simulink model "svpwm_speed"  (R2024b)
settings: Solver=VariableStepAuto  StartTime=0.0  StopTime=inf  RelTol=1e-3
libraries: simulink x2, spsDCVoltageSourceLib x1, spsPermanentMagnetSynchronousMachineLib x1, sldrtlib x1, spsTwoLevelConverterLib x1, spspowerguiLib x1
settings Model: Creator=alienware  LastModifiedBy=20844

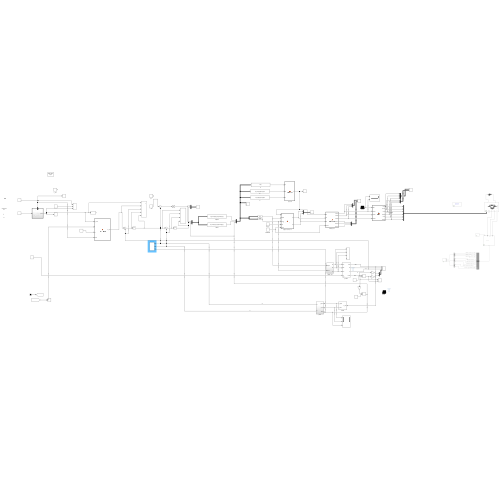
[thumbnail: Simulink's stored preview of the top-level diagram]
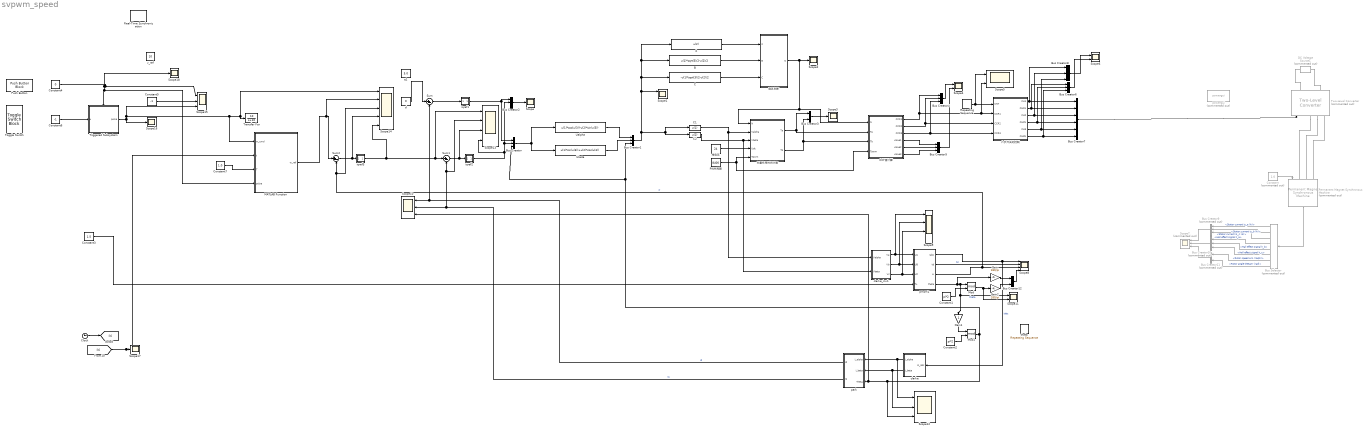
== system svpwm_speed ==
  A : Fcn  Expr=u(2)
  B : Fcn  Expr=u(1)*sqrt(3)/2-u(2)/2
  Bus Creator{,1..2,4..6,8} (7 alike) : BusCreator  Inputs=3
  Bus Creator10 : BusCreator  Commented=on  Inputs=3
  Bus Creator11 : BusCreator  Commented=on  Inputs=2
  Bus Creator12 : BusCreator  Inputs=2
  Bus Creator3 : BusCreator  Inputs=2
  Bus Creator7 : BusCreator  Inputs=6
  Bus Creator9 : BusCreator  Commented=on  Inputs=3
  Bus Selector : BusSelector  Commented=on  OutputSignals=Stator current is_a (A),Stator current is_b (A),Stator current is_c (A),Hall effect signal h_a,Hall effect signal h_b,Hall effect signal h_c,Rotor speed wm (rad/s),Rotor angle thetam (rad)
  C : Fcn  Expr=-u(1)*sqrt(3)/2-u(2)/2
  C1 : Fcn  Expr=u(1)
  C2 : Fcn  Expr=u(2)
  CCR值计算 : MATLAB Function  TreatAsAtomicUnit=on
  Clock : Clock
  Constant : Constant  Commented=on  Value=1.0
  Constant1 : Constant  Value=pi*2
  Constant2 : Constant  Value=pi*2
  Constant3 : Constant  Value=1.5
  Constant4 : Constant  Value=0
  Constant5 : Constant  Value=-1
  Constant6 : Constant  Value=-1
  Constant7 : Constant  Value=1.0
  DC Voltage Source1 : spsDCVoltageSourceLib/DC Voltage Source  Commented=on  Amplitude=24  Measurements=None
  Gain : Gain  Gain=180/pi
  Gain1 : Gain
  Gain2 : Gain  Gain=180/pi
  MATLAB Function : MATLAB Function  TreatAsAtomicUnit=on
  Mod : Math  Operator=mod
  Mod1 : Math  Operator=mod
  PWM周期 : Constant  Value=8400
  Permanent Magnet Synchronous Machine : spsPermanentMagnetSynchronousMachineLib/Permanent Magnet Synchronous Machine  Commented=on  NbPhases=3  FluxDistribution=Sinusoidal  RotorType=Round  MechanicalLoad=Torque Tm  PresetModel=No  ShowDetailedParameters=on  MeasurementBus=off  Resistance=0.0485  Inductance=8.5e-3  dqInductances=[8.5e-3,8.5e-3]  La=0.000395  MachineConstant=Flux linkage established by magnets (V.s)  Flux=0.1194  VoltageCst=86.6271  TorqueCst=0.7164  Flat=120  Mechanical=[0.0027 0.0004924 4 0]  PolePairs=4  InitialConditions=[0,0, 0,0]  InitialConditions5ph=[0 0 0 0 0 0]  RefAngle=Aligned with phase A axis (original Park)  IterativeDiscreteModel=Trapezoidal non iterative  TsBlock=-1  TsPowergui=0
  Push Button : PushButtonBlock  OnValue=2  OffValue=0.000000
  Real-Time Synchronization : sldrtlib/Real-Time Synchronization  SampleTime=0.001  MaxMissedTicks=inf  ShowMissedTicks=off  YieldWhenWaiting=off
  Repeating Sequence : simulink/Sources/Repeating Sequence  rep_seq_t=[0 0.00005 0.0001]  rep_seq_y=[0 4200 0]
  Scope{,2..3,16..18} (6 alike) : Scope
  Scope{1,10,12,15} (4 alike) : Scope  NumInputPorts=3
  Scope{4..6,11} (4 alike) : Scope  NumInputPorts=2
  Scope13 : Scope  NumInputPorts=4
  Scope14 : Scope  NumInputPorts=5
  Scope7 : Scope  Commented=on  NumInputPorts=3
  Scope8 : Scope  NumInputPorts=4
  Scope9 : Scope  NumInputPorts=4
  Sum : Sum  Inputs=|+-
  Sum1 : Sum  Inputs=|+-
  Sum2 : Sum  Inputs=|+-
  Toggle Switch : ToggleSwitchBlock
      settings: Values={{'Off', 'On'}, [-1 1]}
  Transfer Fcn : TransferFcn  Numerator=[10]  Denominator=[1 10]
  Triggered Subsystem : Subsystem  TreatAsAtomicUnit=on
  Two-Level Converter : spsTwoLevelConverterLib/Two-Level Converter  Commented=on  ModelType=Switching devices  Ron=1e-3  Rs=1e6  Cs=inf  Vforward=[0,0]  Ron_Diode=1e-3  Rs_Diode=1e6  Cs_Diode=inf  Vf_Diode=1e-3  Rs_CurrentSource=inf  Ron_ACsource=1e-3
      settings: LibrarySourceBlock=sps_lib/Power Electronics/Two-Level Converter
  Ualpha : Fcn  Expr=u(1)*cos(u(3))-u(2)*sin(u(3))
  Ubeta : Fcn  Expr=u(1)*sin(u(3))+u(2)*cos(u(3))
  clarke : Subsystem
  clarke_inv1 : Subsystem
  d : Constant  Value=0
  iqref1 : Subsystem  mask(PI Controller){I=0, P=0, sat=[-500, 500]}
      mask prompts: I "Integral"; P "Proportional:"; sat "Minimum and maximum outputs:"
      mask init:
      | min=sat(1);max=sat(2);
      mask Display: disp('PI')
  iqref2 : Subsystem  mask(PI Controller){I=0, P=1, sat=[-500, 500]}
      mask prompts: I "Integral"; P "Proportional:"; sat "Minimum and maximum outputs:"
      mask init:
      | min=sat(1);max=sat(2);
      mask Display: disp('PI')
  iqref3 : Subsystem  mask(PI Controller){I=10, P=10, sat=[-100, 100]}
      mask prompts: I "Integral"; P "Proportional:"; sat "Minimum and maximum outputs:"
      mask init:
      | min=sat(1);max=sat(2);
      mask Display: disp('PI')
  park : Subsystem
  pmsm1 : Subsystem  mask(hao){CL=0.175, Pm=4, Ld=0.0085, Lq=0.0085, rs=2.875, J=0.0008}
      mask help: pmsm
      mask Help: no
  powergui : spspowerguiLib/powergui  Priority=1  Commented=on  SimulationMode=Discrete  SampleTime=0.000001  frequency=60  Iterations=50  frequencyindice=0  Pbase=100e6  ErrMax=1e-4  UnitsV=kV  UnitsW=MW  buscounter=0  FunctionMessages=off  echomessages=off  EnableUseOfTLC=off  CurrentSourceSwitches=off  DisableSnubberDevices=off  DisableRonSwitches=off  DisableVfSwitches=off  DisplayEquations=off  AutomaticDiscreteSolvers=off  SolverType=Tustin/Backward Euler (TBE)  Interpol=off  ExternalGateDelay=off  methode=off  Ts=100  x0status=blocks  SPID=on  SwTol=0  HookPort=off  NonlinearTolerance=1e-4  nMaxIteration=100  ContinueOnMaxIteration=off  RestoreLinks=warning  ResistiveCurrentMeasurement=off  Frange=[0:2:500]  Ylog=off  Xlog=on  ShowGrid=off  save=off  variable=ZData  structure=0  ZoomFFT=off  StartTime=0.0  cycles=1  DisplayStyle=1  fundamental=60  FreqAxis=off  MaxFrequency=1000  frequencyindicesteady=1  RmsSteady=1  display=off
  q1 : Constant  Value=5.0
  "theta " : simulink/Sources/Repeating Sequence  rep_seq_t=[0 1]  rep_seq_y=[0 2*pi]
  v_ref : Constant  Value=10
  六步开关的控制 : MATLAB Function  TreatAsAtomicUnit=on
  扇区判断 : MATLAB Function  TreatAsAtomicUnit=on
  矢量作用时间计算 : MATLAB Function  TreatAsAtomicUnit=on
  线电压 : Constant  Value=24
  wires:
  Sum/1 -> iqref1/1(In_1)
  Sum1/1 -> Scope13/3, iqref2/1(In_1)
  Bus Creator/1 -> Ubeta/1, Ualpha/1
  Ualpha/1 -> Bus Creator1/1
  Ubeta/1 -> Bus Creator1/2
  Bus Creator2/1 -> Scope/1
  Bus Creator1/1 -> A/1, B/1, C/1, Scope1/1, C1/1, C2/1
  A/1 -> 扇区判断/1(A)
  B/1 -> 扇区判断/2(B)
  C/1 -> 扇区判断/3(C)
  扇区判断/1(N) -> Scope2/1, CCR值计算/1(N), 矢量作用时间计算/1(N)
  C1/1 -> clarke_inv1/1(Valpha), 矢量作用时间计算/2(Valpha)
  C2/1 -> clarke_inv1/2(Vbeta), 矢量作用时间计算/3(Vbeta)
  线电压/1 -> 矢量作用时间计算/4(Udc)
  PWM周期/1 -> CCR值计算/4(Tpwm), 矢量作用时间计算/5(Tpwm)
  矢量作用时间计算/1(Ta) -> Bus Creator3/1, CCR值计算/2(Ta)
  矢量作用时间计算/2(Tb) -> Bus Creator3/2, CCR值计算/3(Tb)
  Bus Creator3/1 -> Scope3/1
  CCR值计算/3(CCR3) -> 六步开关的控制/4(CCR3), Bus Creator4/3
  CCR值计算/2(CCR2) -> Bus Creator4/2, 六步开关的控制/3(CCR2)
  CCR值计算/1(CCR1) -> Scope5/2, 六步开关的控制/2(CCR1), Bus Creator4/1
  Bus Creator4/1 -> Scope4/1
  CCR值计算/4(value1) -> Bus Creator5/1
  CCR值计算/5(value2) -> Bus Creator5/2
  CCR值计算/6(value3) -> Bus Creator5/3
  Bus Creator5/1 -> Scope4/2
  Repeating Sequence/1 -> 六步开关的控制/1(CNT), Scope5/1
  六步开关的控制/1(CH1) -> Bus Creator7/1, Bus Creator8/1
  六步开关的控制/2(CH1N) -> Bus Creator7/2, Bus Creator6/1
  六步开关的控制/3(CH2) -> Bus Creator7/3, Bus Creator8/2
  六步开关的控制/5(CH3) -> Bus Creator7/5, Bus Creator8/3
  六步开关的控制/4(CH2N) -> Bus Creator7/4, Bus Creator6/2
  六步开关的控制/6(CH3N) -> Bus Creator7/6, Bus Creator6/3
  Bus Creator8/1 -> Scope6/1
  Bus Creator7/1 -> Two-Level Converter/1
  Constant/1 -> Permanent Magnet Synchronous Machine/1
  Permanent Magnet Synchronous Machine/1 -> Bus Selector/1
  Bus Creator9/1 -> Scope7/1
  Bus Creator10/1 -> Scope7/2
  Bus Creator11/1 -> Scope7/3
  Bus Selector/1 -> Bus Creator9/1  "<Stator current is_a (A)>"
  Bus Selector/2 -> Bus Creator9/2  "<Stator current is_b (A)>"
  Bus Selector/3 -> Bus Creator9/3  "<Stator current is_c (A)>"
  Bus Selector/4 -> Bus Creator10/1  "<Hall effect signal h_a>"
  Bus Selector/5 -> Bus Creator10/2  "<Hall effect signal h_b>"
  Bus Selector/6 -> Bus Creator10/3  "<Hall effect signal h_c>"
  Bus Selector/7 -> Bus Creator11/1  "<Rotor speed wm (rad/s)>"
  Bus Selector/8 -> Bus Creator11/2  "<Rotor angle thetam (rad)>"
  Bus Creator6/1 -> Scope6/2
  clarke_inv1/1(Va) -> Scope9/1, pmsm1/1(UA)
  clarke_inv1/2(Vb) -> Scope9/2, pmsm1/2(UB)
  clarke_inv1/3(Vc) -> Scope9/3, pmsm1/3(UC)
  Constant3/1 -> pmsm1/4(TL)
  pmsm1/1(iabc) -> Scope8/1, clarke/1(is_abc)  "iabc"
  pmsm1/2(td) -> Scope8/2  "td"
  pmsm1/3(w) -> Scope8/3, Scope14/3, Sum2/2  "w"
  pmsm1/4(theta) -> Gain/1, Scope11/1, Gain1/1, Mod/1  "theta"
  Constant1/1 -> Mod/2
  Mod/1 -> Gain2/1, Scope11/2
  Gain/1 -> Bus Creator12/1
  clarke/1(I_alpha) -> park/1(I_alpha), Scope12/1
  clarke/2(I_beta) -> park/2(I_beta), Scope12/2
  park/1(Id) -> Sum/2, Scope10/1  "id"
  park/2(Iq) -> Scope13/2, Sum1/2, Scope10/2  "iq"
  Gain1/1 -> Mod1/1
  Constant2/1 -> Mod1/2
  Gain2/1 -> Bus Creator12/2
  Bus Creator12/1 -> Scope8/4
  d/1 -> Sum/1
  iqref3/1(Out_1) -> Scope14/5, Scope13/1, Sum1/1
  iqref1/1(Out_1) -> Bus Creator/1, Bus Creator2/1
  iqref2/1(Out_1) -> Scope13/4, Bus Creator2/2, Bus Creator/2
  Mod1/1 -> Bus Creator/3, Bus Creator1/3, Scope12/3, Scope10/3, park/3(Theta)
  Triggered Subsystem/1(pulse) -> Scope15/3, MATLAB Function/1(w_cmd), Transfer Fcn/1, Scope14/1, Scope16/1
  Sum2/1 -> Scope14/4, iqref3/1(In_1)
  Constant5/1 -> Scope15/2
  Constant6/1 -> Triggered Subsystem/1(u)
  MATLAB Function/1(w_ref) -> Scope14/2, Sum2/1
  Clock/1 -> [t]
  [t] -> MATLAB Function/2(t), Scope17/1
  Constant7/1 -> MATLAB Function/3(T)
  Constant4/1 -> MATLAB Function/4(pulse), Triggered Subsystem/Trigger, Scope18/1, Scope15/1
  connections:
  DC Voltage Source1/RConn1 -- Two-Level Converter/RConn1
  DC Voltage Source1/LConn1 -- Two-Level Converter/RConn2
  Permanent Magnet Synchronous Machine/LConn3 -- Two-Level Converter/LConn3
  Two-Level Converter/LConn2 -- Permanent Magnet Synchronous Machine/LConn2
  Two-Level Converter/LConn1 -- Permanent Magnet Synchronous Machine/LConn1

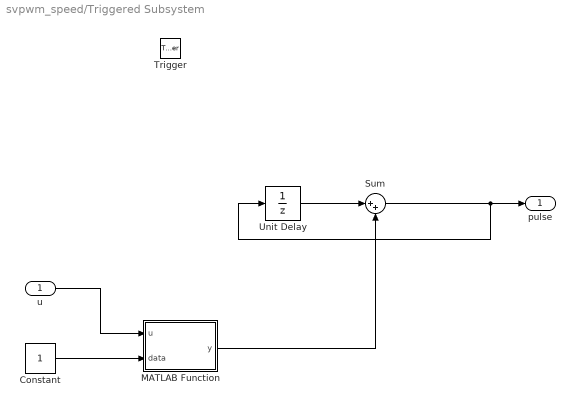
== system svpwm_speed/Triggered Subsystem ==
  u : Inport
  Trigger : TriggerPort  VariantControl=(inherit)
  Constant : Constant
  MATLAB Function : MATLAB Function  TreatAsAtomicUnit=on
  Sum : Sum  Inputs=|++
  Unit Delay : UnitDelay  InitialCondition=10  InputProcessing=Columns as channels (frame based)  SampleTime=-1  HasFrameUpgradeWarning=on
  pulse : Outport
  wires:
  Unit Delay/1 -> Sum/1
  MATLAB Function/1(y) -> Sum/2
  Sum/1 -> Unit Delay/1, pulse/1
  u/1 -> MATLAB Function/1(u)
  Constant/1 -> MATLAB Function/2(data)

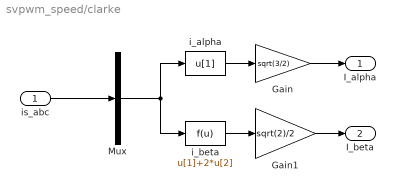
== system svpwm_speed/clarke ==
  is_abc : Inport
  Gain : Gain  Gain=sqrt(3/2)  SaturateOnIntegerOverflow=on  OutDataTypeStr=Inherit: Same as input  ParamDataTypeStr=Inherit: Same as input
  Gain1 : Gain  Gain=sqrt(2)/2  SaturateOnIntegerOverflow=on  OutDataTypeStr=Inherit: Same as input  ParamDataTypeStr=Inherit: Same as input
  Mux : Mux  Inputs=[3]
  i_alpha : Fcn  Expr=u[1]
  i_beta : Fcn  Expr=u[1]+2*u[2]
  I_alpha : Outport  InitialOutput=0
  I_beta : Outport  Port=2  InitialOutput=0
  wires:
  Mux/1 -> i_beta/1, i_alpha/1
  is_abc/1 -> Mux/1
  i_beta/1 -> Gain1/1
  i_alpha/1 -> Gain/1
  Gain/1 -> I_alpha/1
  Gain1/1 -> I_beta/1

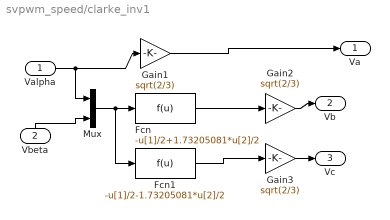
== system svpwm_speed/clarke_inv1 ==
  Valpha : Inport
  Vbeta : Inport  Port=2
  Fcn : Fcn  Expr=-u[1]/2+1.73205081*u[2]/2
  Fcn1 : Fcn  Expr=-u[1]/2-1.73205081*u[2]/2
  Gain1 : Gain  Gain=sqrt(2/3)  SaturateOnIntegerOverflow=on  OutDataTypeStr=Inherit: Same as input  ParamDataTypeStr=Inherit: Same as input
  Gain2 : Gain  Gain=sqrt(2/3)  SaturateOnIntegerOverflow=on  OutDataTypeStr=Inherit: Same as input  ParamDataTypeStr=Inherit: Same as input
  Gain3 : Gain  Gain=sqrt(2/3)  SaturateOnIntegerOverflow=on  OutDataTypeStr=Inherit: Same as input  ParamDataTypeStr=Inherit: Same as input
  Mux : Mux  Inputs=2
  Va : Outport
  Vb : Outport  Port=2
  Vc : Outport  Port=3
  wires:
  Gain3/1 -> Vc/1
  Gain2/1 -> Vb/1
  Gain1/1 -> Va/1
  Vbeta/1 -> Mux/2
  Valpha/1 -> Mux/1, Gain1/1
  Fcn1/1 -> Gain3/1
  Fcn/1 -> Gain2/1
  Mux/1 -> Fcn1/1, Fcn/1

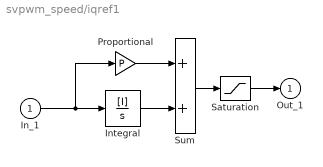
== system svpwm_speed/iqref1 ==
  In_1 : Inport
  Integral : TransferFcn  Numerator=[I]  Denominator=[1 0]
  Proportional : Gain  Gain=P  SaturateOnIntegerOverflow=on  OutDataTypeStr=Inherit: Same as input  ParamDataTypeStr=Inherit: Same as input
  Saturation : Saturate  UpperLimit=max  LowerLimit=min
  Sum : Sum  InputSameDT=on  SaturateOnIntegerOverflow=on  OutDataTypeStr=Inherit: Same as first input
  Out_1 : Outport  InitialOutput=0
  wires:
  Saturation/1 -> Out_1/1
  Sum/1 -> Saturation/1
  Proportional/1 -> Sum/1
  In_1/1 -> Proportional/1, Integral/1
  Integral/1 -> Sum/2

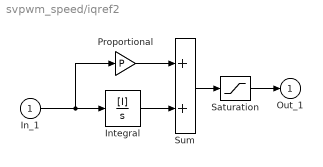
== system svpwm_speed/iqref2 ==
  In_1 : Inport
  Integral : TransferFcn  Numerator=[I]  Denominator=[1 0]
  Proportional : Gain  Gain=P  SaturateOnIntegerOverflow=on  OutDataTypeStr=Inherit: Same as input  ParamDataTypeStr=Inherit: Same as input
  Saturation : Saturate  UpperLimit=max  LowerLimit=min
  Sum : Sum  InputSameDT=on  SaturateOnIntegerOverflow=on  OutDataTypeStr=Inherit: Same as first input
  Out_1 : Outport  InitialOutput=0
  wires:
  Integral/1 -> Sum/2
  In_1/1 -> Integral/1, Proportional/1
  Proportional/1 -> Sum/1
  Sum/1 -> Saturation/1
  Saturation/1 -> Out_1/1

== system svpwm_speed/iqref3 ==
  In_1 : Inport
  Integral : TransferFcn  Numerator=[I]  Denominator=[1 0]
  Proportional : Gain  Gain=P  SaturateOnIntegerOverflow=on  OutDataTypeStr=Inherit: Same as input  ParamDataTypeStr=Inherit: Same as input
  Saturation : Saturate  UpperLimit=max  LowerLimit=min
  Sum : Sum  InputSameDT=on  SaturateOnIntegerOverflow=on  OutDataTypeStr=Inherit: Same as first input
  Out_1 : Outport  InitialOutput=0
  wires:
  Integral/1 -> Sum/2
  In_1/1 -> Integral/1, Proportional/1
  Proportional/1 -> Sum/1
  Sum/1 -> Saturation/1
  Saturation/1 -> Out_1/1

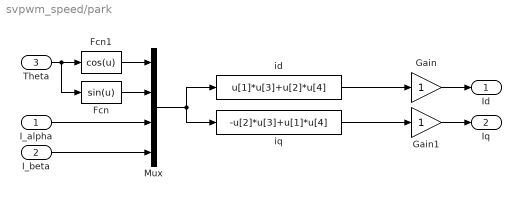
== system svpwm_speed/park ==
  I_alpha : Inport
  I_beta : Inport  Port=2
  Theta : Inport  Port=3
  Fcn : Fcn  Expr=sin(u)
  Fcn1 : Fcn  Expr=cos(u)
  Gain : Gain  SaturateOnIntegerOverflow=on  OutDataTypeStr=Inherit: Same as input  ParamDataTypeStr=Inherit: Same as input
  Gain1 : Gain  SaturateOnIntegerOverflow=on  OutDataTypeStr=Inherit: Same as input  ParamDataTypeStr=Inherit: Same as input
  Mux : Mux  Inputs=[1 1 1 1]
  id : Fcn  Expr=u[1]*u[3]+u[2]*u[4]
  iq : Fcn  Expr=-u[2]*u[3]+u[1]*u[4]
  Id : Outport  InitialOutput=0
  Iq : Outport  Port=2  InitialOutput=0
  wires:
  Fcn/1 -> Mux/2
  Fcn1/1 -> Mux/1
  Theta/1 -> Fcn1/1, Fcn/1
  Mux/1 -> iq/1, id/1
  I_alpha/1 -> Mux/3
  iq/1 -> Gain1/1
  id/1 -> Gain/1
  Gain/1 -> Id/1
  Gain1/1 -> Iq/1
  I_beta/1 -> Mux/4

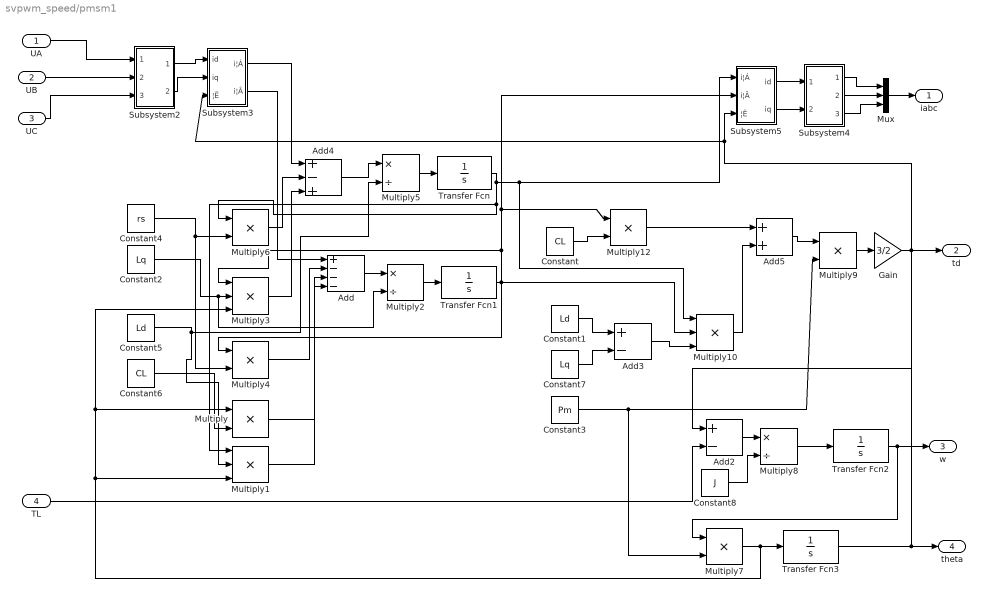
== system svpwm_speed/pmsm1 ==
  UA : Inport
  UB : Inport  Port=2
  UC : Inport  Port=3
  TL : Inport  Port=4
  Add : Sum  Inputs=+---  SaturateOnIntegerOverflow=on  OutDataTypeStr=Inherit: Same as first input
  Add2 : Sum  Inputs=+-  InputSameDT=on  SaturateOnIntegerOverflow=on  OutDataTypeStr=Inherit: Same as first input
  Add3 : Sum  Inputs=+-  InputSameDT=on  SaturateOnIntegerOverflow=on  OutDataTypeStr=Inherit: Same as first input
  Add4 : Sum  Inputs=+-+  InputSameDT=on  SaturateOnIntegerOverflow=on  OutDataTypeStr=Inherit: Same as first input
  Add5 : Sum  InputSameDT=on  SaturateOnIntegerOverflow=on  OutDataTypeStr=Inherit: Same as first input
  Constant : Constant  Value=CL
  Constant1 : Constant  Value=Ld
  Constant2 : Constant  Value=Lq
  Constant3 : Constant  Value=Pm
  Constant4 : Constant  Value=rs
  Constant5 : Constant  Value=Ld
  Constant6 : Constant  Value=CL
  Constant7 : Constant  Value=Lq
  Constant8 : Constant  Value=J
  Gain : Gain  Gain=3/2  SaturateOnIntegerOverflow=on  OutDataTypeStr=Inherit: Same as input  ParamDataTypeStr=Inherit: Same as input
  Multiply{,4,6..7,9,12} (6 alike) : Product  Inputs=**  SaturateOnIntegerOverflow=on  OutDataTypeStr=Inherit: Same as first input
  Multiply1 : Product  Inputs=***  SaturateOnIntegerOverflow=on  OutDataTypeStr=Inherit: Same as first input
  Multiply10 : Product  Inputs=***  SaturateOnIntegerOverflow=on  OutDataTypeStr=Inherit: Same as first input
  Multiply2 : Product  Inputs=*/  SaturateOnIntegerOverflow=on  OutDataTypeStr=Inherit: Same as first input
  Multiply3 : Product  Inputs=***  SaturateOnIntegerOverflow=on  OutDataTypeStr=Inherit: Same as first input
  Multiply5 : Product  Inputs=*/  SaturateOnIntegerOverflow=on  OutDataTypeStr=Inherit: Same as first input
  Multiply8 : Product  Inputs=*/  SaturateOnIntegerOverflow=on  OutDataTypeStr=Inherit: Same as first input
  Mux : Mux  Inputs=3
  Subsystem2 : Subsystem  mask(hao){}
      mask help: 3/2
      mask Help: no
      mask Display: disp('3/2')
  Subsystem3 : Subsystem  mask(2/2){}
      mask help: qdtoMT
      mask Help: none
  Subsystem4 : Subsystem  mask(hao){}
      mask help: 2/3
      mask Help: npi
      mask Display: disp('2/3')
  Subsystem5 : Subsystem  mask(2/2){}
      mask help: mt-todq
      mask Help: no
  Transfer Fcn : TransferFcn  Denominator=[1 0]  AbsoluteTolerance=1e-3
  Transfer Fcn1 : TransferFcn  Denominator=[1 0]
  Transfer Fcn2 : TransferFcn  Denominator=[1 0]
  Transfer Fcn3 : TransferFcn  Denominator=[1 0]
  iabc : Outport
  td : Outport  Port=2
  w : Outport  Port=3
  theta : Outport  Port=4
  wires:
  UB/1 -> Subsystem2/2(In2)
  UA/1 -> Subsystem2/1(In1)
  Subsystem4/2(Out2) -> Mux/2
  Subsystem4/1(Out1) -> Mux/1
  Gain/1 -> Add2/1, td/1
  Transfer Fcn3/1 -> theta/1, Subsystem3/3(¦Ë), Subsystem5/3(¦Ë)
  UC/1 -> Subsystem2/3(In3)
  Multiply8/1 -> Transfer Fcn2/1
  Mux/1 -> iabc/1
  Subsystem4/3(Out3) -> Mux/3
  Multiply9/1 -> Gain/1
  Add5/1 -> Multiply9/1
  Transfer Fcn2/1 -> w/1, Multiply7/1
  Add3/1 -> Multiply10/3
  Constant/1 -> Multiply12/2
  Multiply7/1 -> Multiply1/3, Multiply/1, Multiply3/3, Transfer Fcn3/1
  Constant6/1 -> Multiply/2
  Constant5/1 -> Multiply5/2, Multiply1/2
  Constant2/1 -> Multiply2/2, Multiply3/2
  Transfer Fcn1/1 -> Subsystem5/2(i¦Â), Multiply12/1, Multiply3/1, Multiply10/2, Multiply4/1
  Constant4/1 -> Multiply4/2, Multiply6/2
  Transfer Fcn/1 -> Subsystem5/1(i¦Á), Multiply10/1, Multiply1/1, Multiply6/1
  Subsystem2/1(Out1) -> Subsystem3/1(id)
  Subsystem2/2(Out2) -> Subsystem3/2(iq)
  Subsystem3/1(i¦Á) -> Add4/1
  Multiply6/1 -> Add4/2
  Multiply3/1 -> Add4/3
  Add4/1 -> Multiply5/1
  Subsystem3/2(i¦Â) -> Add/1
  Add/1 -> Multiply2/1
  Multiply4/1 -> Add/2
  Multiply/1 -> Add/3
  Multiply1/1 -> Add/4
  Constant1/1 -> Add3/1
  Constant7/1 -> Add3/2
  Multiply12/1 -> Add5/1
  Multiply10/1 -> Add5/2
  Constant3/1 -> Multiply9/2, Multiply7/2
  Subsystem5/1(id) -> Subsystem4/1(In1)
  Subsystem5/2(iq) -> Subsystem4/2(In3)
  Add2/1 -> Multiply8/1
  Constant8/1 -> Multiply8/2
  TL/1 -> Add2/2
  Multiply5/1 -> Transfer Fcn/1
  Multiply2/1 -> Transfer Fcn1/1

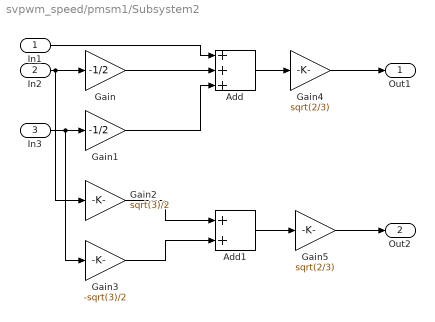
== system svpwm_speed/pmsm1/Subsystem2 ==
  In1 : Inport
  In2 : Inport  Port=2
  In3 : Inport  Port=3
  Add : Sum  Inputs=+++  InputSameDT=on  SaturateOnIntegerOverflow=on  OutDataTypeStr=Inherit: Same as first input
  Add1 : Sum  InputSameDT=on  SaturateOnIntegerOverflow=on  OutDataTypeStr=Inherit: Same as first input
  Gain : Gain  Gain=-1/2  SaturateOnIntegerOverflow=on  OutDataTypeStr=Inherit: Same as input  ParamDataTypeStr=Inherit: Same as input
  Gain1 : Gain  Gain=-1/2  SaturateOnIntegerOverflow=on  OutDataTypeStr=Inherit: Same as input  ParamDataTypeStr=Inherit: Same as input
  Gain2 : Gain  Gain=sqrt(3)/2  SaturateOnIntegerOverflow=on  OutDataTypeStr=Inherit: Same as input  ParamDataTypeStr=Inherit: Same as input
  Gain3 : Gain  Gain=-sqrt(3)/2  SaturateOnIntegerOverflow=on  OutDataTypeStr=Inherit: Same as input  ParamDataTypeStr=Inherit: Same as input
  Gain4 : Gain  Gain=sqrt(2/3)  SaturateOnIntegerOverflow=on  OutDataTypeStr=Inherit: Same as input  ParamDataTypeStr=Inherit: Same as input
  Gain5 : Gain  Gain=sqrt(2/3)  SaturateOnIntegerOverflow=on  OutDataTypeStr=Inherit: Same as input  ParamDataTypeStr=Inherit: Same as input
  Out1 : Outport
  Out2 : Outport  Port=2
  wires:
  Gain/1 -> Add/2
  Gain1/1 -> Add/3
  Gain2/1 -> Add1/1
  Gain3/1 -> Add1/2
  In1/1 -> Add/1
  Add/1 -> Gain4/1
  In2/1 -> Gain/1, Gain2/1
  In3/1 -> Gain1/1, Gain3/1
  Add1/1 -> Gain5/1
  Gain4/1 -> Out1/1
  Gain5/1 -> Out2/1

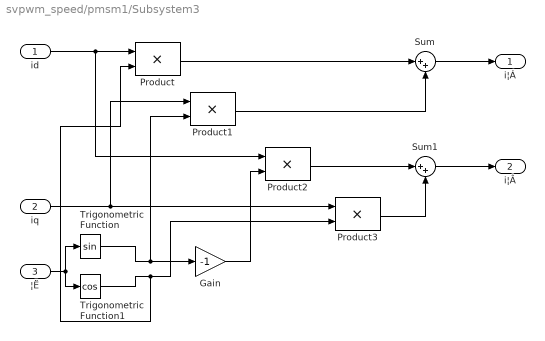
== system svpwm_speed/pmsm1/Subsystem3 ==
  id : Inport
  iq : Inport  Port=2
  ¦Ë : Inport  Port=3
  Gain : Gain  Gain=-1  SaturateOnIntegerOverflow=on  OutDataTypeStr=Inherit: Same as input  ParamDataTypeStr=Inherit: Same as input
  Product{,1..3} (4 alike) : Product  SaturateOnIntegerOverflow=on  OutDataTypeStr=Inherit: Same as first input
  Sum : Sum  Inputs=|++  InputSameDT=on  SaturateOnIntegerOverflow=on  OutDataTypeStr=Inherit: Same as first input
  Sum1 : Sum  Inputs=|++  InputSameDT=on  SaturateOnIntegerOverflow=on  OutDataTypeStr=Inherit: Same as first input
  Trigonometric Function : Trigonometry
  Trigonometric Function1 : Trigonometry  Operator=cos
  i¦Á : Outport
  i¦Â : Outport  Port=2
  wires:
  id/1 -> Product2/1, Product/1
  Product/1 -> Sum/1
  Sum/1 -> i¦Á/1
  Product2/1 -> Sum1/1
  Sum1/1 -> i¦Â/1
  iq/1 -> Product1/1, Product3/1
  ¦Ë/1 -> Trigonometric Function/1, Trigonometric Function1/1
  Trigonometric Function1/1 -> Product3/2, Product/2
  Trigonometric Function/1 -> Gain/1, Product1/2
  Gain/1 -> Product2/2
  Product1/1 -> Sum/2
  Product3/1 -> Sum1/2

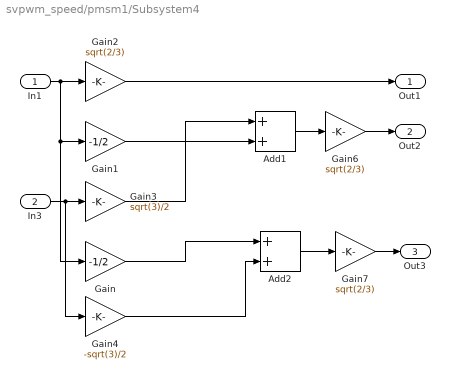
== system svpwm_speed/pmsm1/Subsystem4 ==
  In1 : Inport
  In3 : Inport  Port=2
  Add1 : Sum  InputSameDT=on  SaturateOnIntegerOverflow=on  OutDataTypeStr=Inherit: Same as first input
  Add2 : Sum  InputSameDT=on  SaturateOnIntegerOverflow=on  OutDataTypeStr=Inherit: Same as first input
  Gain : Gain  Gain=-1/2  SaturateOnIntegerOverflow=on  OutDataTypeStr=Inherit: Same as input  ParamDataTypeStr=Inherit: Same as input
  Gain1 : Gain  Gain=-1/2  SaturateOnIntegerOverflow=on  OutDataTypeStr=Inherit: Same as input  ParamDataTypeStr=Inherit: Same as input
  Gain2 : Gain  Gain=sqrt(2/3)  SaturateOnIntegerOverflow=on  OutDataTypeStr=Inherit: Same as input  ParamDataTypeStr=Inherit: Same as input
  Gain3 : Gain  Gain=sqrt(3)/2  SaturateOnIntegerOverflow=on  OutDataTypeStr=Inherit: Same as input  ParamDataTypeStr=Inherit: Same as input
  Gain4 : Gain  Gain=-sqrt(3)/2  SaturateOnIntegerOverflow=on  OutDataTypeStr=Inherit: Same as input  ParamDataTypeStr=Inherit: Same as input
  Gain6 : Gain  Gain=sqrt(2/3)  SaturateOnIntegerOverflow=on  OutDataTypeStr=Inherit: Same as input  ParamDataTypeStr=Inherit: Same as input
  Gain7 : Gain  Gain=sqrt(2/3)  SaturateOnIntegerOverflow=on  OutDataTypeStr=Inherit: Same as input  ParamDataTypeStr=Inherit: Same as input
  Out1 : Outport
  Out2 : Outport  Port=2
  Out3 : Outport  Port=3
  wires:
  Gain1/1 -> Add1/1
  Gain3/1 -> Add1/2
  Gain/1 -> Add2/1
  Gain4/1 -> Add2/2
  Add1/1 -> Gain6/1
  Add2/1 -> Gain7/1
  In1/1 -> Gain2/1, Gain1/1, Gain/1
  Gain2/1 -> Out1/1
  Gain6/1 -> Out2/1
  In3/1 -> Gain3/1, Gain4/1
  Gain7/1 -> Out3/1

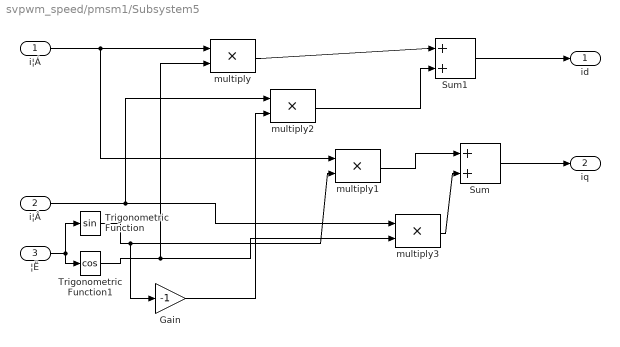
== system svpwm_speed/pmsm1/Subsystem5 ==
  i¦Á : Inport
  i¦Â : Inport  Port=2
  ¦Ë : Inport  Port=3
  Gain : Gain  Gain=-1  SaturateOnIntegerOverflow=on  OutDataTypeStr=Inherit: Same as input  ParamDataTypeStr=Inherit: Same as input
  Sum : Sum  Inputs=|++  SaturateOnIntegerOverflow=on  OutDataTypeStr=Inherit: Same as first input
  Sum1 : Sum  Inputs=|++  SaturateOnIntegerOverflow=on  OutDataTypeStr=Inherit: Same as first input
  Trigonometric Function : Trigonometry
  Trigonometric Function1 : Trigonometry  Operator=cos
  multiply{,1..3} (4 alike) : Product  SaturateOnIntegerOverflow=on  OutDataTypeStr=Inherit: Same as first input
  id : Outport
  iq : Outport  Port=2
  wires:
  Gain/1 -> multiply2/2
  Trigonometric Function/1 -> Gain/1, multiply1/2
  Trigonometric Function1/1 -> multiply/2, multiply3/2
  multiply3/1 -> Sum/2
  multiply2/1 -> Sum1/2
  i¦Â/1 -> multiply3/1, multiply2/1
  multiply1/1 -> Sum/1
  i¦Á/1 -> multiply/1, multiply1/1
  Sum/1 -> iq/1
  Sum1/1 -> id/1
  multiply/1 -> Sum1/1
  ¦Ë/1 -> Trigonometric Function1/1, Trigonometric Function/1

== matlab function svpwm_speed/矢量作用时间计算 ==
  data: N input; Valpha input; Ta output; Vbeta input; Udc input; Tpwm input; Tb output
function [Ta,Tb] =VectorCalculate(N,Valpha,Vbeta,Udc,Tpwm )
Ta=double(0);
Tb=double(0);

X=(sqrt(3)*Tpwm)/Udc*Vbeta;
Y=(sqrt(3)*Tpwm)/Udc*((sqrt(3)/2)*Valpha-(1/2)*Vbeta);
Z=(sqrt(3)*Tpwm)/Udc*(-(sqrt(3)/2)*Valpha-(1/2)*Vbeta);

if N==3 %1%
    Ta=Y;
    Tb=X;

end
if N==1 %2%
    Ta=-Y;
    Tb=-Z;

end
if N==5 %3%
    Ta=X;
    Tb=Z;

end
if N==4 %4% 
    Ta=-X;
    Tb=-Y;

end
if N==6 %5%
    Ta=Z;
    Tb=Y;

end
if N==2 %6%
    Ta=-Z;
    Tb=-X;

end

== matlab function svpwm_speed/扇区判断 ==
  data: A input; N output; B input; C input
function N =SectorJudge(A,B,C)


N=0;
if A>0
    N=N+1;
end
if B>0
    N=N+2; 
end
if C>0
    N=N+4;
end

== matlab function svpwm_speed/CCR值计算 ==
  data: N input; Ta input; CCR1 output; Tb input; CCR2 output; CCR3 output; Tpwm input; value1 output; value2 output; value3 output
function [CCR1,CCR2,CCR3,value1,value2,value3] =CCRCalculate(N,Ta,Tb,Tpwm)
CCR1=double(0);
CCR2=double(0);
CCR3=double(0);
Ttemp=Ta+Tb;
if Ttemp>Tpwm
    Ta=Ta/Ttemp*Tpwm;
    Tb=Tb/Ttemp*Tpwm;
end
value1=(Tpwm-Ta-Tb)/4.0;
value2=value1+Ta/2.0;
value3=value2+Tb/2.0;
switch (N)
    case 3
        CCR1= value1;
        CCR2= value2;
        CCR3= value3;
     case 1
        CCR1= value2;
        CCR2= value1;
        CCR3= value3;
     case 5
        CCR1= value3 ;
        CCR2= value1;
        CCR3= value2;
     case 4
        CCR1= value3;
        CCR2= value2;
        CCR3= value1;
     case 6
        CCR1= value2;
        CCR2= value3;
        CCR3= value1;
     case 2
        CCR1= value1;
        CCR2= value3;
        CCR3= value2;
end

== matlab function svpwm_speed/六步开关的控制 ==
  data: CNT input; CCR1 input; CH1 output; CH1N output; CCR2 input; CH2 output; CH2N output; CH3 output; CCR3 input; CH3N output
function [CH1,CH1N,CH2,CH2N,CH3,CH3N] =PWM(CNT,CCR1,CCR2,CCR3)
if CNT<CCR1
    CH1=0;
    CH1N=1;
else
    CH1=1;
    CH1N=0;
end
if CNT<CCR2
    CH2=0;
    CH2N=1;
else
    CH2=1;
    CH2N=0;
end
if CNT<CCR3
    CH3=0;
    CH3N=1;
else
    CH3=1;
    CH3N=0;
end

== matlab function svpwm_speed/Triggered Subsystem/MATLAB Function ==
  data: u input; y output; data input
function y = fcn(u, data)

y=0;
if u>0
    y=data;
end
if u<0
    y=-1*data;
end
if u==0
    y=0;
end

== matlab function svpwm_speed/MATLAB Function ==
  settings: updateMethod=DISCRETE
  data: w_cmd input; t input; T input; w_ref output; pulse input
function w_ref = s_curve_speed(w_cmd, t, T, pulse)
% w_cmd: 阶梯目标速度
% t: Clock(秒)
% T: 过渡时间(秒)，例如 3
% pulse: 上升沿单脉冲(按一下=1个采样周期的1)

persistent w0 wf t0
if isempty(t0)
    w0 = w_cmd;
    wf = w_cmd;
    t0 = t;
end

% 用当前段参数先算“此刻的平滑输出”
w_now = minjerk_5th(w0, wf, t, T, t0);

% 阶跃/按键触发：更新 w0/wf/t0
if pulse ~= 0
    w0 = w_now;   % 新起点 = 当前平滑输出
    wf = w_cmd;   % 新终点 = 新阶梯目标
    t0 = t;       % 新起始时刻
    w_ref = w0;   % 触发这一拍输出起点
else
    w_ref = w_now;
end
end

function w = minjerk_5th(w0, wf, t, T, t0)
dt = t - t0;

if dt <= 0
    w = w0;
    return;
elseif dt >= T
    w = wf;
    return;
end

s = dt / T; % 0~1
h = 10*s^3 - 15*s^4 + 6*s^5;
w = w0 + (wf - w0) * h;
end
